simulink model "F16sim_trim"  (R2023b)
settings: Solver=ode4  StartTime=0  StopTime=0.5  FixedStep=0.005  RelTol=1e-3  EnableMultiTasking=on
values from neighbouring files (symbols this model uses):
  U_trim = Zstar(10:13)    [DOTRIM.m]    (also in trimcond.mat = [0.153996989097 -0.694820589342 -0.00017032672875 0.00137758)
  X_trim = [Zstar(1:9); 0; 0; 0; x13]    [DOTRIM.m]    (also in trimcond.mat = [501.999994561 0.0505398298476 9.15927892863e-06 -3.32783191)
  xcg = 0.35    [DOTRIM.m]    (also in trimcond.mat)
settings Model: Creator=keviczky  LastModifiedBy=suvo
settings DataIOCC: Decimation=50  SaveFormat=Array  SignalLoggingSaveFormat=ModelDataLogs  ReturnWorkspaceOutputs=off  SignalLoggingName=sigsOut
settings OptimizationCC: BooleanDataType=off
settings DebuggingCC: SaveWithParameterizedLinksMsg=none  UnderspecifiedInitializationDetection=Classic  MergeDetectMultiDrivingBlocksExec=none  SignalResolutionControl=TryResolveAllWithWarning  MultiTaskDSMMsg=warning  MultiTaskCondExecSysMsg=none  UnconnectedInputMsg=warning  UnconnectedOutputMsg=warning  UnconnectedLineMsg=warning
settings HardwareCC: ProdBitPerPointer=32  ProdBitPerSizeT=32  ProdBitPerPtrDiffT=32  ProdLargestAtomicFloat=None  ProdIntDivRoundTo=Undefined  ProdEndianess=Unspecified  ProdWordSize=32  ProdHWDeviceType=32-bit Generic  TargetUnknown=on
settings ModelReferenceCC: PropagateSignalLabelsOutOfModel=off
settings GRTTargetCC: CombineOutputUpdateFcns=off  GRTInterface=on
settings ConfigComp: CovMetricSettings=dw  CovSaveCumulativeToWorkspaceVar=on  CovSaveSingleToWorkspaceVar=on

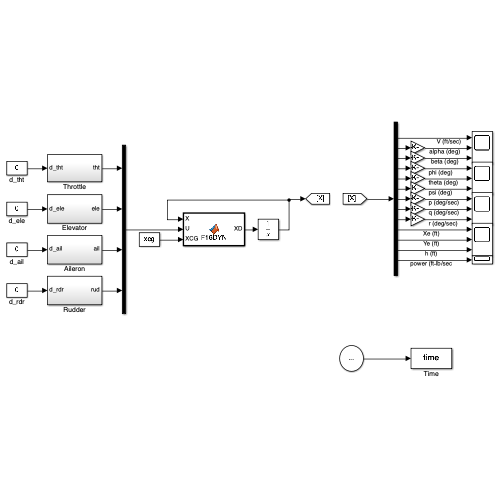
[thumbnail: Simulink's stored preview of the top-level diagram]
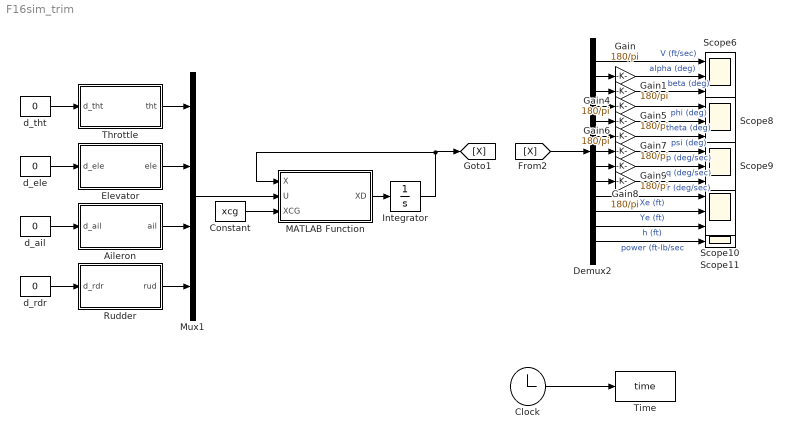
== system F16sim_trim ==
  Aileron : Subsystem
  Clock : Clock
  Constant : Constant  Value=xcg
  Demux2 : Demux  Outputs=13
  Elevator : Subsystem
  Gain{,1,4..9} (8 alike) : Gain  Gain=180/pi
  Integrator : Integrator  InitialCondition=X_trim
  MATLAB Function : MATLAB Function  TreatAsAtomicUnit=on
  Mux1 : Mux
  Rudder : Subsystem
  Scope{6,8..10} (4 alike) : Scope  NumInputPorts=3
  Scope11 : Scope
  Throttle : Subsystem
  Time : ToWorkspace  VariableName=time  SampleTime=-1
      settings: Decimation=100
  d_ail : Constant  Value=0
  d_ele : Constant  Value=0
  d_rdr : Constant  Value=0
  d_tht : Constant  Value=0
  wires:
  Clock/1 -> Time/1
  Throttle/1(tht) -> Mux1/1
  Elevator/1(ele) -> Mux1/2
  Aileron/1(ail) -> Mux1/3
  Rudder/1(rud) -> Mux1/4
  d_tht/1 -> Throttle/1(d_tht)
  d_ele/1 -> Elevator/1(d_ele)
  d_ail/1 -> Aileron/1(d_ail)
  d_rdr/1 -> Rudder/1(d_rdr)
  MATLAB Function/1(XD) -> Integrator/1
  Integrator/1 -> [X], MATLAB Function/1(X)
  Mux1/1 -> MATLAB Function/2(U)
  Demux2/1 -> Scope6/1  "V (ft/sec)"
  Demux2/2 -> Gain/1
  Demux2/3 -> Gain1/1
  Constant/1 -> MATLAB Function/3(XCG)
  Gain/1 -> Scope6/2  "alpha (deg)"
  Gain1/1 -> Scope6/3  "beta (deg)"
  [X] -> Demux2/1
  Demux2/4 -> Gain4/1
  Demux2/5 -> Gain5/1
  Demux2/6 -> Gain6/1
  Gain4/1 -> Scope8/1  "phi (deg)"
  Gain5/1 -> Scope8/2  "theta (deg)"
  Gain6/1 -> Scope8/3  "psi (deg)"
  Demux2/9 -> Gain9/1
  Demux2/8 -> Gain8/1
  Demux2/7 -> Gain7/1
  Gain7/1 -> Scope9/1  "p (deg/sec)"
  Gain8/1 -> Scope9/2  "q (deg/sec)"
  Gain9/1 -> Scope9/3  "r (deg/sec)"
  Demux2/10 -> Scope10/1  "Xe (ft)"
  Demux2/11 -> Scope10/2  "Ye (ft)"
  Demux2/12 -> Scope10/3  "h (ft)"
  Demux2/13 -> Scope11/1  "power (ft-lb/sec"

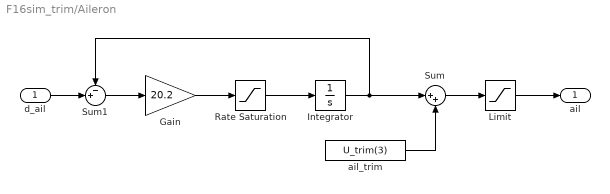
== system F16sim_trim/Aileron ==
  d_ail : Inport
  Gain : Gain  Gain=20.2  SaturateOnIntegerOverflow=on  OutDataTypeStr=Inherit: Same as input  ParamDataTypeStr=Inherit: Same as input
  Integrator : Integrator  UpperSaturationLimit=25  LowerSaturationLimit=-25
  Limit : Saturate  UpperLimit=25  LowerLimit=-25
  Rate Saturation : Saturate  UpperLimit=60  LowerLimit=-60
  Sum : Sum  Inputs=|++  InputSameDT=on  SaturateOnIntegerOverflow=on  OutDataTypeStr=Inherit: Same as first input
  Sum1 : Sum  Inputs=-+|  InputSameDT=on  SaturateOnIntegerOverflow=on  OutDataTypeStr=Inherit: Same as first input
  ail_trim : Constant  Value=U_trim(3)
  ail : Outport
  wires:
  Sum1/1 -> Gain/1
  Gain/1 -> Rate Saturation/1
  Rate Saturation/1 -> Integrator/1
  Integrator/1 -> Sum/1, Sum1/1
  Sum/1 -> Limit/1
  Limit/1 -> ail/1
  ail_trim/1 -> Sum/2
  d_ail/1 -> Sum1/2

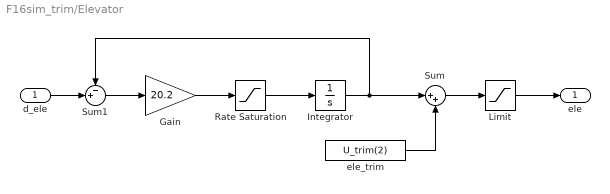
== system F16sim_trim/Elevator ==
  d_ele : Inport
  Gain : Gain  Gain=20.2  SaturateOnIntegerOverflow=on  OutDataTypeStr=Inherit: Same as input  ParamDataTypeStr=Inherit: Same as input
  Integrator : Integrator  UpperSaturationLimit=25  LowerSaturationLimit=-25
  Limit : Saturate  UpperLimit=25  LowerLimit=-25
  Rate Saturation : Saturate  UpperLimit=60  LowerLimit=-60
  Sum : Sum  Inputs=|++  InputSameDT=on  SaturateOnIntegerOverflow=on  OutDataTypeStr=Inherit: Same as first input
  Sum1 : Sum  Inputs=-+|  InputSameDT=on  SaturateOnIntegerOverflow=on  OutDataTypeStr=Inherit: Same as first input
  ele_trim : Constant  Value=U_trim(2)
  ele : Outport
  wires:
  Sum1/1 -> Gain/1
  Gain/1 -> Rate Saturation/1
  Rate Saturation/1 -> Integrator/1
  Integrator/1 -> Sum/1, Sum1/1
  Sum/1 -> Limit/1
  Limit/1 -> ele/1
  ele_trim/1 -> Sum/2
  d_ele/1 -> Sum1/2

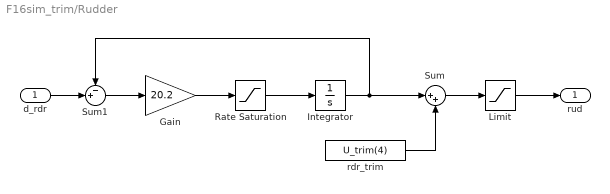
== system F16sim_trim/Rudder ==
  d_rdr : Inport
  Gain : Gain  Gain=20.2  SaturateOnIntegerOverflow=on  OutDataTypeStr=Inherit: Same as input  ParamDataTypeStr=Inherit: Same as input
  Integrator : Integrator  UpperSaturationLimit=25  LowerSaturationLimit=-25
  Limit : Saturate  UpperLimit=25  LowerLimit=-25
  Rate Saturation : Saturate  UpperLimit=60  LowerLimit=-60
  Sum : Sum  Inputs=|++  InputSameDT=on  SaturateOnIntegerOverflow=on  OutDataTypeStr=Inherit: Same as first input
  Sum1 : Sum  Inputs=-+|  InputSameDT=on  SaturateOnIntegerOverflow=on  OutDataTypeStr=Inherit: Same as first input
  rdr_trim : Constant  Value=U_trim(4)
  rud : Outport
  wires:
  Sum1/1 -> Gain/1
  Gain/1 -> Rate Saturation/1
  Rate Saturation/1 -> Integrator/1
  Integrator/1 -> Sum/1, Sum1/1
  Sum/1 -> Limit/1
  Limit/1 -> rud/1
  rdr_trim/1 -> Sum/2
  d_rdr/1 -> Sum1/2

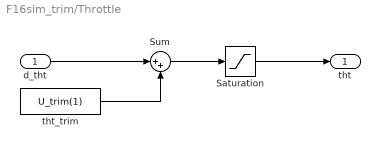
== system F16sim_trim/Throttle ==
  d_tht : Inport
  Saturation : Saturate  UpperLimit=1  LowerLimit=0
  Sum : Sum  Inputs=|++  InputSameDT=on  SaturateOnIntegerOverflow=on  OutDataTypeStr=Inherit: Same as first input
  tht_trim : Constant  Value=U_trim(1)
  tht : Outport
  wires:
  Sum/1 -> Saturation/1
  Saturation/1 -> tht/1
  d_tht/1 -> Sum/1
  tht_trim/1 -> Sum/2

== matlab function F16sim_trim/MATLAB Function ==
  data: X input; U input; XD output; XCG input
function XD = F16DYN(X,U,XCG)
% f16 dynamics

% Author: Subhabrata Ganguli
%
% Ref: Stevens, Brian L.; Lewis, Frank L.; Johnson, Eric N.. 
% Aircraft Control and Simulation: Dynamics, 
% Controls Design, and Autonomous Systems. 
% Wiley.

%% Parameters

AXX = 9496.0;
AYY = 55814.0;
AZZ = 63100.0;
AXZ =   982.0;

AXZS = AXZ^2;
XPQ  = AXZ * (AXX - AYY + AZZ);
GAM = AXX * AZZ - AXZ^2;

XQR = AZZ * (AZZ - AYY) + AXZS;
ZPQ =(AXX-AYY) * AXX + AXZS;
YPR = AZZ - AXX;

WEIGHT = 25000.0;
GD = 32.174;
MASS = WEIGHT/GD;

S = 300;
B = 30;
CBAR = 11.32;
XCGR = 0.35;
HX = 160;
RTOD = 180/pi;

%% Assign State and Control Variables

VT = X(1); 
ALPHA = X(2)*RTOD; 
BETA = X(3)*RTOD;
PHI = X(4); 
THETA = X(5); 
PSI = X(6);
P = X(7); 
Q = X(8); 
R = X(9); 
ALT = X(12); 
POW = X(13);

THTL = U(1);
EL = U(2);
AIL = U(3);
RDR = U(4);

XD = zeros(13,1);

%% Air data computer and engine model

[TFAC, T, RHO, AMACH, QBAR, PS ] = ADC (VT, ALT);
CPOW = TGEAR(THTL);

XD(13) = PDOT(POW,CPOW);     
T = THRUST(POW,ALT,AMACH);

%% Look-up tables and component buildup

CXT = CX (ALPHA,EL);
CYT = CY (BETA,AIL,RDR);
CZT = CZ (ALPHA,BETA,EL);
      
DAIL= AIL/20.0; DRDR= RDR/30.0;

DLDA_OUT = DLDA(ALPHA,BETA);
DLDR_OUT = DLDR(ALPHA,BETA);
DNDA_OUT = DNDA(ALPHA,BETA);
DNDR_OUT = DNDR(ALPHA,BETA);

CLT = CL(ALPHA,BETA) + DLDA_OUT*DAIL + DLDR_OUT*DRDR;
CMT = CM(ALPHA,EL);
CNT = CN(ALPHA,BETA) + DNDA_OUT*DAIL + DNDR_OUT*DRDR;

%% Add damping derivatives

TVT = 0.5/VT; 
B2V = B*TVT; 
CQ = CBAR*Q*TVT;

D = DAMP(ALPHA);

CXT = CXT + CQ * D(1);
CYT = CYT + B2V * ( D(2)*R + D(3)*P );
CZT = CZT + CQ * D(4);
CLT = CLT + B2V * ( D(5)*R + D(6)*P );
CMT = CMT + CQ * D(7) + CZT * (XCGR-XCG);
CNT = CNT + B2V*(D(8)*R + D(9)*P) - CYT*(XCGR-XCG) * CBAR/B;

%% Get ready for state equations

CBTA  = cos(X(3)); 
U     = VT*cos(X(2))*CBTA;
V     = VT * sin(X(3)); 
W     = VT*sin(X(2))*CBTA;
STH   = sin(THETA); 
CTH   = cos(THETA);   
SPH   = sin(PHI);
CPH   = cos(PHI); 
SPSI  = sin(PSI);    
CPSI  = cos(PSI);
QS    = QBAR * S; 
QSB   = QS * B;        
RMQS  = QS/MASS;
GCTH  = GD * CTH; 
QSPH  = Q * SPH;
AY    = RMQS*CYT; 
AZ    = RMQS * CZT;

%% Force Equations

UDOT   = R*V - Q*W - GD*STH + (QS * CXT + T)/MASS;
VDOT   = P*W - R*U + GCTH * SPH + AY;
WDOT   = Q*U - P*V + GCTH * CPH + AZ;
    
DUM   = (U*U + W*W);
XD(1) = (U*UDOT + V*VDOT + W*WDOT)/VT;
XD(2) = (U*WDOT - W*UDOT) / DUM;
XD(3) = (VT*VDOT- V*XD(1)) * CBTA / DUM;

%% Kinematics

XD(4) = P + (STH/CTH)*(QSPH + R*CPH);
XD(5) = Q*CPH - R*SPH;
XD(6) = (QSPH + R*CPH)/CTH;

%% Moments

ROLL  = QSB*CLT;
PITCH = QS *CBAR*CMT;
YAW   = QSB*CNT;
PQ    = P*Q;
QR    = P*R;
QHX   = Q*HX;
XD(7) = ( XPQ*PQ - XQR*QR + AZZ*ROLL + AXZ*(YAW + QHX) )/GAM;
XD(8) = ( YPR*P*R - AXZ*(P^2 - R^2) + PITCH - R*HX )/AYY;
XD(9) = ( ZPQ*PQ - XPQ*QR + AXZ*ROLL + AXX*(YAW + QHX) )/GAM;

%% Navigation

T1 = SPH * CPSI; 
T2 = CPH * STH; 
T3 = SPH * SPSI;
S1 = CTH * CPSI; 
S2 = CTH * SPSI; 
S3 = T1 * STH - CPH * SPSI;
S4 = T3 * STH + CPH * CPSI; 
S5 = SPH * CTH; 
S6 = T2 * CPSI + T3;
S7 = T2 * SPSI - T1; 
S8 = CPH * CTH;

XD(10)  = U * S1 + V * S3 + W * S6;   %   North speed
XD(11)  = U * S2 + V * S4 + W * S7;   %   East speed
XD(12)  = U * STH -V * S5 - W * S8;   %   Vertical speed

XD = XD(:);

end
